simulink model "control_core"  (R2022b)
settings: Solver=VariableStepAuto  StartTime=0.0  StopTime=10.0  RelTol=1e-3
values from neighbouring files (symbols this model uses):
  g = [0, 0, 1]    [myMeasurementFcn.m]    (also in test_DELETE.m = [0,0,0,1])
undefined symbols (not defined in the file or in its folder): airframe
libraries: simulink_extras x2, vrlib x2, aerolibutil x1, sharedtransform x1
settings Model: Creator=aaron  LastModifiedBy=aaron

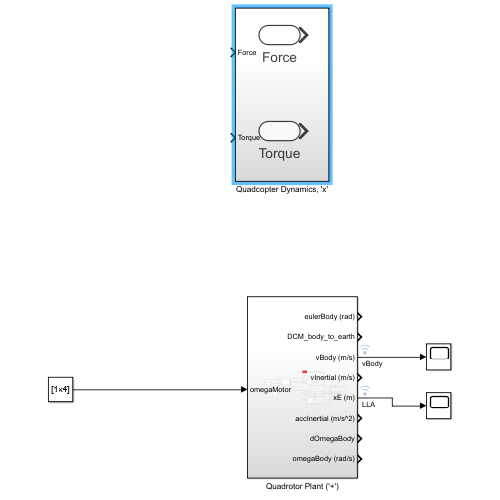
[thumbnail: Simulink's stored preview of the top-level diagram]
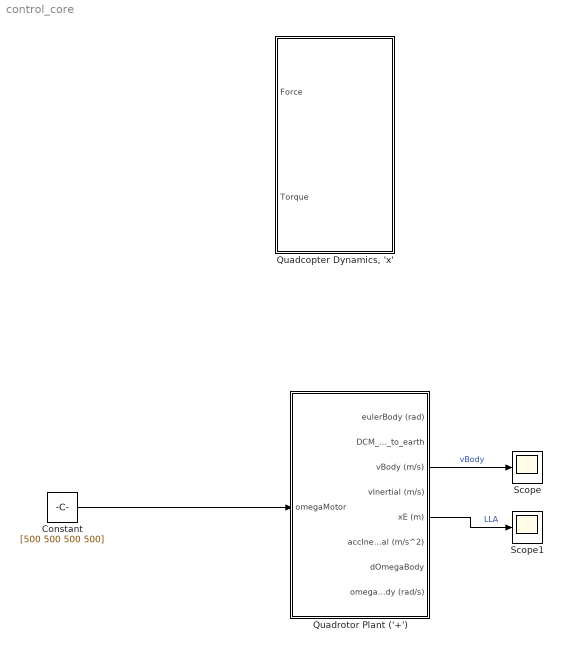
== system control_core ==
  Constant : Constant  Value=[500 500 500 500]
  "Quadcopter Dynamics, 'x'" : Subsystem
  Quadrotor Plant ('+') : Subsystem
  Scope : Scope
  Scope1 : Scope
  wires:
  Constant/1 -> Quadrotor Plant ('+')/1(omegaMotor)
  Quadrotor Plant ('+')/3(vBody (m/s)) -> Scope/1  "vBody"
  Quadrotor Plant ('+')/5(xE (m)) -> Scope1/1  "LLA"

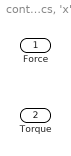
== system control_core/Quadcopter Dynamics, 'x' ==
  Force : Inport
  Torque : Inport  Port=2

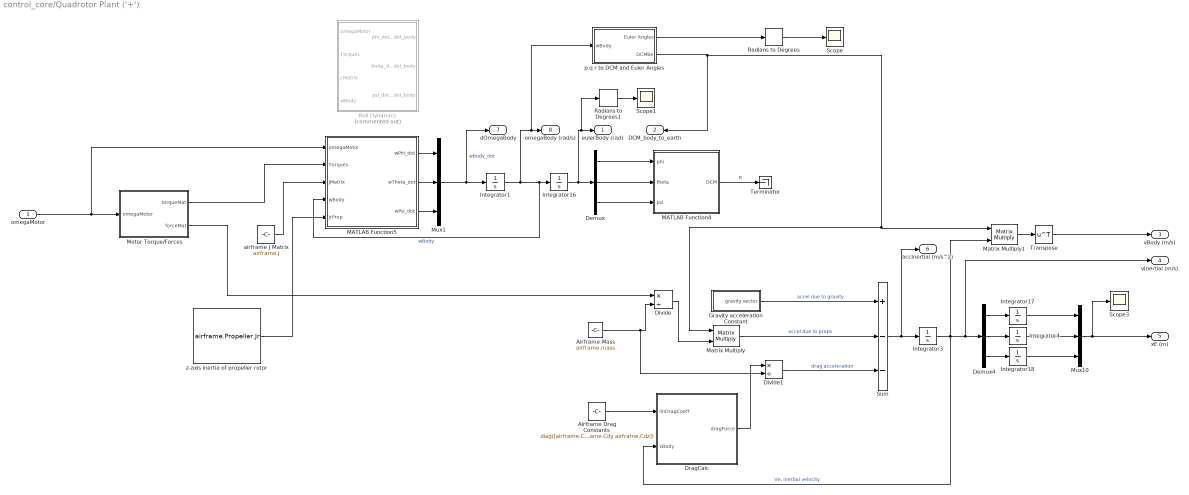
== system control_core/Quadrotor Plant ('+') ==
  omegaMotor : Inport
  Airframe Drag Constants : Constant  Value=diag([airframe.Cdx airframe.Cdy airframe.Cdz])
  Airframe Mass : Constant  Value=airframe.mass
  Demux : Demux  Outputs=3
  Demux4 : Demux  Outputs=3
  Divide : Product  Inputs=*/
  Divide1 : Product  Inputs=*/
  DragCalc : Subsystem
  Gravity acceleration Constant : Subsystem
  Integrator1 : Integrator  InitialCondition=[0 0 0]
  Integrator16 : Integrator  WrapState=on
  Integrator17 : Integrator
  Integrator18 : Integrator  LimitOutput=on  UpperSaturationLimit=0
  Integrator3 : Integrator
  Integrator4 : Integrator
  MATLAB Function4 : MATLAB Function  TreatAsAtomicUnit=on
  MATLAB Function5 : MATLAB Function  TreatAsAtomicUnit=on
  Matrix Multiply : Product  Multiplication=Matrix(*)
  Matrix Multiply1 : Product  Multiplication=Matrix(*)
  Motor Torque/Forces : Subsystem
  Mux1 : Mux  Inputs=3
  Mux10 : Mux  Inputs=3
  Radians to Degrees : simulink_extras/Transformations/Radians to Degrees
  Radians to Degrees1 : simulink_extras/Transformations/Radians to Degrees
  Roll Dynamics : Subsystem  Commented=on
  Scope : Scope
  Scope1 : Scope
  Scope3 : Scope
  Sum : Sum  Inputs=+--
  Terminator : Terminator
  Transpose : Math  Operator=transpose
  airframe J Matrix : Constant  Value=airframe.J
  p q r to DCM and Euler Angles : Subsystem
  z-axis inertia of propeller rotor : Constant  Value=airframe.Propeller.Jr
  eulerBody (rad) : Outport
  DCM_body_to_earth : Outport  Port=2
  vBody (m/s) : Outport  Port=3
  vInertial (m/s) : Outport  Port=4
  xE (m) : Outport  Port=5
  accInertial (m/s^2) : Outport  Port=6
  dOmegaBody : Outport  Port=7
  omegaBody (rad/s) : Outport  Port=8
  wires:
  Motor Torque/Forces/1(torqueMat) -> MATLAB Function5/2(Torques)
  omegaMotor/1 -> MATLAB Function5/1(omegaMotor), Motor Torque/Forces/1(omegaMotor)
  Integrator1/1 -> p q r to DCM and Euler Angles/1(wBody), omegaBody (rad/s)/1, MATLAB Function5/4(wBody), Integrator16/1  "wBody"
  Motor Torque/Forces/2(forceMat) -> Divide/1
  Airframe Mass/1 -> Divide1/2, Divide/2
  Divide/1 -> Matrix Multiply/2
  Matrix Multiply/1 -> Sum/2  "accel due to props"
  Gravity acceleration Constant/1(gravity vector) -> Sum/1  "accel due to gravity"
  DragCalc/1(dragForce) -> Divide1/1
  Sum/1 -> Integrator3/1, accInertial (m/s^2)/1
  Integrator3/1 -> Matrix Multiply1/2, vInertial (m/s)/1, Demux4/1, DragCalc/2(vBody)  "Ve, inertial velocity"
  Airframe Drag Constants/1 -> DragCalc/1(linDragCoeff)
  Matrix Multiply1/1 -> Transpose/1
  Mux10/1 -> Scope3/1, xE (m)/1
  Mux1/1 -> dOmegaBody/1, Integrator1/1  "wBody_dot"
  Demux/1 -> MATLAB Function4/1(phi)
  Demux/2 -> MATLAB Function4/2(theta)
  Demux/3 -> MATLAB Function4/3(psi)
  Integrator16/1 -> Demux/1, Radians to Degrees1/1, eulerBody (rad)/1
  Demux4/1 -> Integrator17/1
  Demux4/2 -> Integrator4/1
  Demux4/3 -> Integrator18/1
  Integrator4/1 -> Mux10/2
  Integrator17/1 -> Mux10/1
  p q r to DCM and Euler Angles/1(Euler Angles) -> Radians to Degrees/1
  airframe J Matrix/1 -> MATLAB Function5/3(JMatrix)
  MATLAB Function5/1(wPhi_dot) -> Mux1/1
  MATLAB Function5/2(wTheta_dot) -> Mux1/2
  MATLAB Function5/3(wPsi_dot) -> Mux1/3
  z-axis inertia of propeller rotor/1 -> MATLAB Function5/5(JrProp)
  Transpose/1 -> vBody (m/s)/1
  Radians to Degrees/1 -> Scope/1
  p q r to DCM and Euler Angles/2(DCMbe) -> Matrix Multiply/1, Matrix Multiply1/1, DCM_body_to_earth/1
  MATLAB Function4/1(DCM) -> Terminator/1  "R"
  Radians to Degrees1/1 -> Scope1/1
  Integrator18/1 -> Mux10/3
  Divide1/1 -> Sum/3  "drag acceleration"

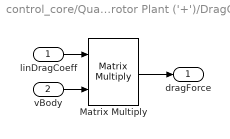
== system control_core/Quadrotor Plant ('+')/DragCalc ==
  linDragCoeff : Inport
  vBody : Inport  Port=2
  Matrix Multiply : Product  Multiplication=Matrix(*)
  dragForce : Outport
  wires:
  linDragCoeff/1 -> Matrix Multiply/1
  vBody/1 -> Matrix Multiply/2
  Matrix Multiply/1 -> dragForce/1

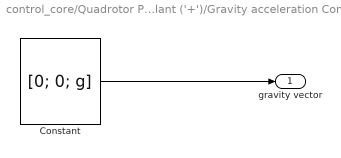
== system control_core/Quadrotor Plant ('+')/Gravity acceleration Constant ==
  Constant : Constant  Value=[0; 0; g]
  gravity vector : Outport
  wires:
  Constant/1 -> gravity vector/1

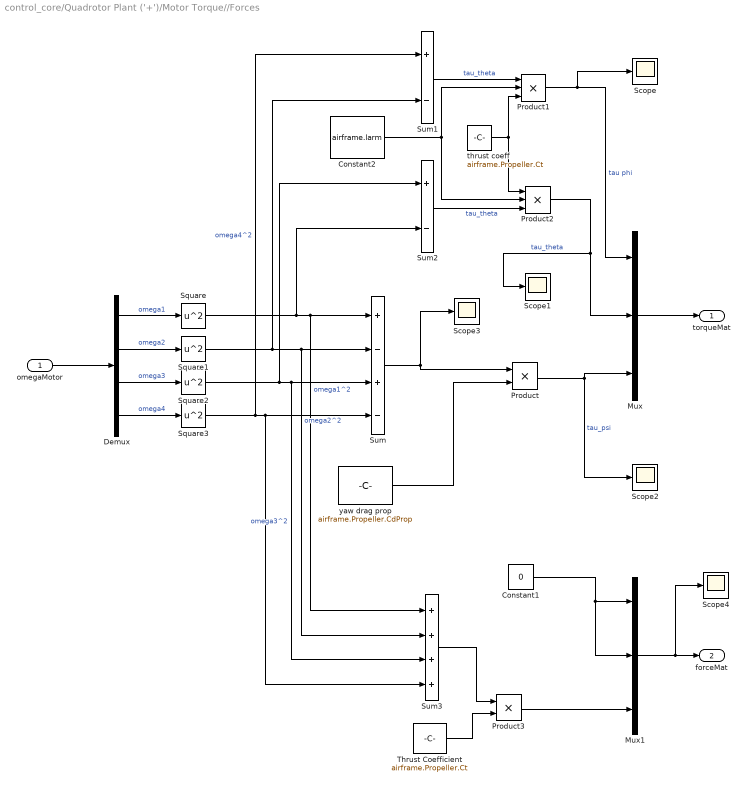
== system control_core/Quadrotor Plant ('+')/Motor Torque//Forces ==
  omegaMotor : Inport
  Constant1 : Constant  Value=0
  Constant2 : Constant  Value=airframe.larm
  Demux : Demux
  Mux : Mux  Inputs=3
  Mux1 : Mux  Inputs=3
  Product : Product
  Product1 : Product  Inputs=3
  Product2 : Product  Inputs=3
  Product3 : Product
  Scope{,1..4} (5 alike) : Scope
  Square{,1..3} (4 alike) : Math  Operator=square
  Sum : Sum  Inputs=+-+-
  Sum1 : Sum  Inputs=+-
  Sum2 : Sum  Inputs=+-
  Sum3 : Sum  Inputs=++++
  Thrust Coefficient : Constant  Value=airframe.Propeller.Ct
  thrust coeff : Constant  Value=airframe.Propeller.Ct
  yaw drag prop : Constant  Value=airframe.Propeller.CdProp
  torqueMat : Outport
  forceMat : Outport  Port=2
  wires:
  omegaMotor/1 -> Demux/1
  Demux/1 -> Square/1  "omega1"
  Demux/2 -> Square1/1  "omega2"
  Demux/3 -> Square2/1  "omega3"
  Demux/4 -> Square3/1  "omega4"
  Square2/1 -> Sum2/1, Sum3/3, Sum/3  "omega3^2"
  Square1/1 -> Sum1/2, Sum3/2, Sum/2  "omega2^2"
  Square/1 -> Sum2/2, Sum3/1, Sum/1  "omega1^2"
  Square3/1 -> Sum1/1, Sum3/4, Sum/4  "omega4^2"
  Sum/1 -> Scope3/1, Product/1
  Product/1 -> Mux/3, Scope2/1  "tau_psi"
  yaw drag prop/1 -> Product/2
  Product2/1 -> Mux/2, Scope1/1  "tau_theta"
  Product1/1 -> Scope/1, Mux/1  "tau phi"
  Constant2/1 -> Product2/2, Product1/2
  Sum1/1 -> Product1/1  "tau_theta"
  Mux/1 -> torqueMat/1
  Sum3/1 -> Product3/1
  Thrust Coefficient/1 -> Product3/2
  Mux1/1 -> Scope4/1, forceMat/1
  Product3/1 -> Mux1/3
  Constant1/1 -> Mux1/2, Mux1/1
  Sum2/1 -> Product2/3  "tau_theta"
  thrust coeff/1 -> Product1/3, Product2/1

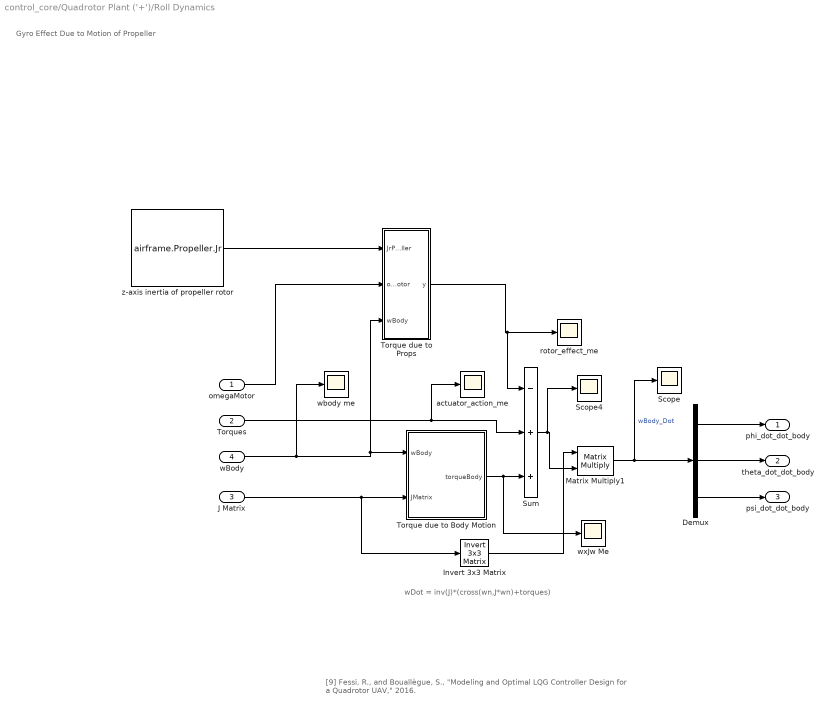
== system control_core/Quadrotor Plant ('+')/Roll Dynamics ==
  note: Gyro Effect Due to Motion of Propeller
  note: [9] Fessi, R., and Bouallègue, S., "Modeling and Optimal LQG Controller Design for a Quadrotor UAV," 2016.
  note: wDot = inv(J)*(cross(wn,J*wn)+torques)
  omegaMotor : Inport
  Torques : Inport  Port=2
  J Matrix : Inport  Port=3
  wBody : Inport  Port=4
  Demux : Demux  Outputs=3
  Invert 3x3 Matrix : aerolibutil/Invert  3x3 Matrix
  Matrix Multiply1 : Product  Multiplication=Matrix(*)
  Scope : Scope
  Scope4 : Scope
  Sum : Sum  Inputs=-++
  Torque due to Body Motion : Subsystem
  Torque due to Props : Subsystem
  actuator_action_me : Scope
  rotor_effect_me : Scope
  wbody me : Scope
  wxJw Me : Scope
  z-axis inertia of propeller rotor : Constant  Value=airframe.Propeller.Jr
  phi_dot_dot_body : Outport
  theta_dot_dot_body : Outport  Port=2
  psi_dot_dot_body : Outport  Port=3
  wires:
  wBody/1 -> wbody me/1, Torque due to Props/3(wBody), Torque due to Body Motion/1(wBody)
  J Matrix/1 -> Invert 3x3 Matrix/1, Torque due to Body Motion/2(JMatrix)
  Invert 3x3 Matrix/1 -> Matrix Multiply1/1
  Sum/1 -> Scope4/1, Matrix Multiply1/2
  Matrix Multiply1/1 -> Scope/1, Demux/1  "wBody_Dot"
  Demux/1 -> phi_dot_dot_body/1
  Demux/2 -> theta_dot_dot_body/1
  Demux/3 -> psi_dot_dot_body/1
  Torques/1 -> actuator_action_me/1, Sum/2
  z-axis inertia of propeller rotor/1 -> Torque due to Props/1(JrPropeller)
  omegaMotor/1 -> Torque due to Props/2(omegaMotor)
  Torque due to Props/1(y) -> Sum/1, rotor_effect_me/1
  Torque due to Body Motion/1(torqueBody) -> wxJw Me/1, Sum/3

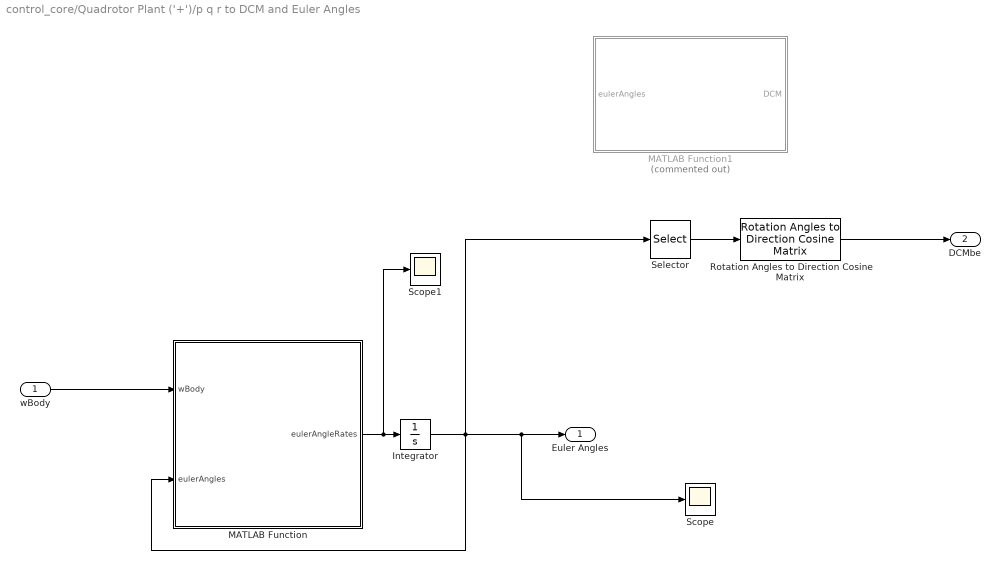
== system control_core/Quadrotor Plant ('+')/p q r to DCM and Euler Angles ==
  wBody : Inport
  Integrator : Integrator  WrapState=on
  MATLAB Function : MATLAB Function  TreatAsAtomicUnit=on
  MATLAB Function1 : MATLAB Function  Commented=on  TreatAsAtomicUnit=on
  Rotation Angles to Direction Cosine Matrix : sharedtransform/Rotation Angles to Direction Cosine Matrix  rotationOrder=ZYX  aMode=aMode
  Scope : Scope
  Scope1 : Scope
  Selector : Selector  InputPortWidth=3  IndexOptions=Index vector (dialog)  Indices=[3 2 1]  OutputSizes=1
  Euler Angles : Outport
  DCMbe : Outport  Port=2
  wires:
  wBody/1 -> MATLAB Function/1(wBody)
  MATLAB Function/1(eulerAngleRates) -> Scope1/1, Integrator/1
  Selector/1 -> Rotation Angles to Direction Cosine Matrix/1
  Integrator/1 -> Selector/1, Scope/1, Euler Angles/1, MATLAB Function/2(eulerAngles)
  Rotation Angles to Direction Cosine Matrix/1 -> DCMbe/1

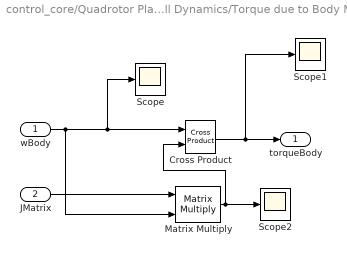
== system control_core/Quadrotor Plant ('+')/Roll Dynamics/Torque due to Body Motion ==
  wBody : Inport
  JMatrix : Inport  Port=2
  Cross Product : vrlib/Utilities/Cross Product
  Matrix Multiply : Product  Multiplication=Matrix(*)
  Scope : Scope
  Scope1 : Scope
  Scope2 : Scope
  torqueBody : Outport
  wires:
  Matrix Multiply/1 -> Cross Product/2, Scope2/1
  wBody/1 -> Matrix Multiply/2, Scope/1, Cross Product/1
  JMatrix/1 -> Matrix Multiply/1
  Cross Product/1 -> Scope1/1, torqueBody/1

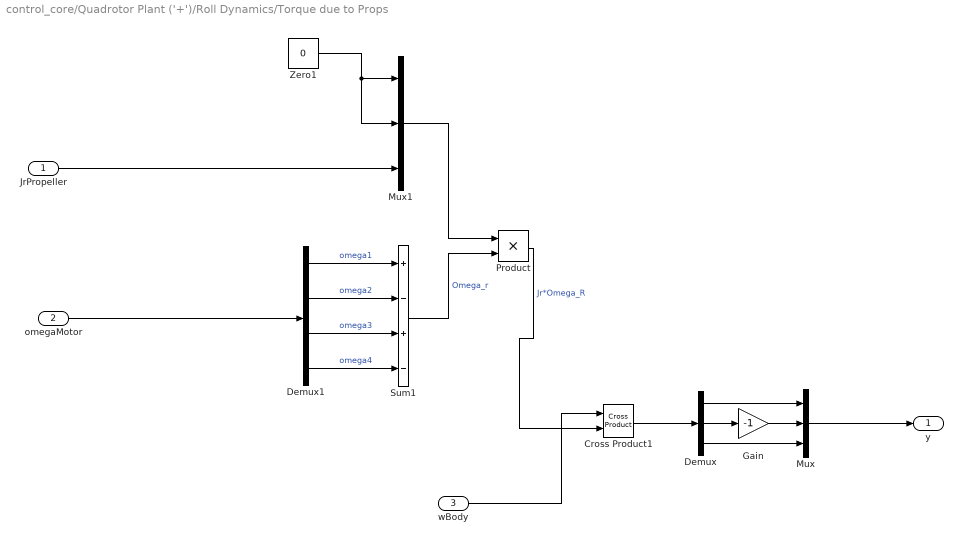
== system control_core/Quadrotor Plant ('+')/Roll Dynamics/Torque due to Props ==
  JrPropeller : Inport
  omegaMotor : Inport  Port=2
  wBody : Inport  Port=3
  Cross Product1 : vrlib/Utilities/Cross Product
  Demux : Demux  Outputs=3
  Demux1 : Demux
  Gain : Gain  Gain=-1
  Mux : Mux  Inputs=3
  Mux1 : Mux  Inputs=3
  Product : Product
  Sum1 : Sum  Inputs=+-+-
  Zero1 : Constant  Value=0  OutDataTypeStr=Inherit: Inherit via back propagation
  y : Outport
  wires:
  Demux1/1 -> Sum1/1  "omega1"
  Demux1/2 -> Sum1/2  "omega2"
  Zero1/1 -> Mux1/2, Mux1/1
  Demux1/4 -> Sum1/4  "omega4"
  Product/1 -> Cross Product1/2  "Jr*Omega_R"
  Sum1/1 -> Product/2  "Omega_r"
  Demux1/3 -> Sum1/3  "omega3"
  Mux1/1 -> Product/1
  JrPropeller/1 -> Mux1/3
  wBody/1 -> Cross Product1/1
  omegaMotor/1 -> Demux1/1
  Cross Product1/1 -> Demux/1
  Mux/1 -> y/1
  Demux/1 -> Mux/1
  Demux/2 -> Gain/1
  Gain/1 -> Mux/2
  Demux/3 -> Mux/3

== matlab function control_core/Quadrotor Plant ('+')/p q r to DCM and Euler Angles/MATLAB Function ==
  data: wBody input; eulerAngleRates output; eulerAngles input
function eulerAngleRates = fcn(wBody,eulerAngles)

% Inertial frame angular velocities
phi = eulerAngles(1);
theta = eulerAngles(2);
psi = eulerAngles(3);
p = wBody(1);
q = wBody(2);
r = wBody(3);

rotMat = [1 sin(phi)*tan(theta) cos(phi)*tan(theta);
    0 cos(phi) -sin(phi);
    0 sin(phi)/cos(theta) cos(phi)/cos(theta)];
eulerAngleRates = rotMat*wBody;

% phidot = p+(q*sin(phi)+r*cos(phi))*tan(theta);
% thetadot = q*cos(phi)-r*sin(phi);
% psidot = (q*sin(phi)+r*cos(phi))/cos(theta);


% eulerAngleRates = [phidot;thetadot;psidot];


% rotBodytoInertial = [1 sin(phi)*sin(theta)/cos(theta) cos(phi)*sin(theta)/cos(theta);
%     0 cos(phi) -sin(phi);
%     0 sin(phi)/cos(theta) cos(phi)/cos(theta)];
% 
% eulerAngleRates = rotBodytoInertial*wBody;

== matlab function control_core/Quadrotor Plant ('+')/p q r to DCM and Euler Angles/MATLAB Function1 ==
  data: eulerAngles input; DCM output
function DCM = fcn(eulerAngles)

phi = eulerAngles(1);
theta = eulerAngles(2);
psi = eulerAngles(3);


DCM = [cos(psi)*cos(phi)-cos(theta)*sin(phi)*sin(psi), cos(psi)*sin(phi)+cos(theta)*cos(phi)*sin(psi), sin(psi)*sin(theta);
    -sin(psi)*cos(phi)-cos(theta)*sin(phi)*cos(psi) -sin(psi)*sin(phi)+cos(theta)*cos(phi)*cos(psi) cos(psi)*sin(theta);
    sin(theta)*sin(phi) -sin(theta)*cos(phi) cos(theta)];

== matlab function control_core/Quadrotor Plant ('+')/MATLAB Function4 ==
  data: DCM output; phi input; theta input; psi input
function DCM = DCM_body_to_inertial(phi,theta,psi)

% Performs a ZYX roation to rotate from body to inertial coordinate frame
% 
DCM = [cos(theta)*cos(psi), cos(theta)*sin(psi), -sin(theta);...
    -sin(psi)*cos(phi)+sin(theta)*sin(phi)*cos(psi), cos(psi)*cos(phi)+sin(phi)*sin(theta)*sin(psi), sin(phi)*cos(theta);...
    sin(phi)*sin(psi)+cos(phi)*sin(theta)*cos(psi), -sin(phi)*cos(psi)+cos(phi)*sin(theta)*sin(psi), cos(theta)*cos(phi)];
    

DCM = DCM';

% % % Trans_mat1=[(cos(psi)*cos(theta)), (-sin(psi)*cos(phi)+cos(psi)*sin(theta)*sin(phi)), (sin(psi)*sin(phi)+cos(psi)*sin(theta)*cos(phi));...
% % %           (sin(psi)*cos(theta)), (cos(psi)*cos(phi)+sin(theta)*sin(psi)*sin(phi)), (-cos(psi)*sin(phi)+sin(theta)*sin(psi)*cos(phi));...
% % %           (-sin(theta)), (cos(theta)*sin(phi)), (cos(theta)*cos(phi))];
% % %       
% % % 
% % % 
% % % R_phi=[1, 0, 0;...
% % %        0, cos(phi), sin(phi);...
% % %        0, -sin(phi), cos(phi)];
% % %    
% % % R_theta=[cos(theta), 0, -sin(theta);...
% % %         0, 1, 0;...
% % %         sin(theta), 0, cos(theta)];
% % % 
% % % R_psi=[cos(psi), sin(psi), 0;...
% % %        -sin(psi), cos(psi), 0;...
% % %        0, 0, 1];
% % %    
% % %   Trans_mat= R_psi*R_theta*R_phi;
% % %   DCM=Trans_mat;

== matlab function control_core/Quadrotor Plant ('+')/MATLAB Function5 ==
  data: omegaMotor input; wPhi_dot output; Torques input; JMatrix input; wBody input; JrProp input; wTheta_dot output; wPsi_dot output
function [wPhi_dot,wTheta_dot,wPsi_dot] = fcn(omegaMotor,Torques,JMatrix,wBody,JrProp)

Ixx = JMatrix(1,1);
Iyy = JMatrix(2,2);
Izz = JMatrix(3,3);

wPhi = wBody(1);
wTheta = wBody(2);
wPsi = wBody(3);

omegaR = omegaMotor(1)-omegaMotor(2)+omegaMotor(3)-omegaMotor(4);

wPhi_dot = ((Iyy-Izz)*wTheta*wPsi+JrProp*omegaR*wTheta+Torques(1))/Ixx;
wTheta_dot = ((Izz-Ixx)*wPhi*wPsi-JrProp*omegaR*wPhi+Torques(2))/Iyy;
wPsi_dot = ((Ixx-Iyy)*wTheta*wPhi+Torques(3))/Izz;
